simulink model "Scenario_1"  (R2020b)
settings: Solver=ode1  StartTime=0.0  StopTime=10  FixedStep=Ts  RelTol=1e-3
InitFcn:
  | Scenario_1_parameters;
values from neighbouring files (symbols this model uses):
  c0 = c0_zeb    (= 6.57988e-09)    [Scenario_17_parameters.m]    (also in Scenario_1_parameters.m = 6.37282e-09; Scenario_2_parameters.m = 6.37282e-09; Scenario_3_parameters.m)
  c1 = c1_zeb    (= 9.15905e-09)    [Scenario_17_parameters.m]    (also in Scenario_1_parameters.m = 8.76156e-09; Scenario_2_parameters.m = 8.76156e-09; Scenario_3_parameters.m)
  fg = 50    [Scenario_17_parameters.m]    (also in Scenario_1_parameters.m; Scenario_2_parameters.m; Scenario_3_parameters.m)
  G1gen = 0.50    (= 0.5)    [Scenario_17_parameters.m]    (also in Scenario_1_parameters.m = 0.2; Scenario_2_parameters.m = 0.1245; Scenario_3_parameters.m = 0.45)
  G2gen = 0.30    (= 0.3)    [Scenario_1_parameters.m]    (also in Scenario_2_parameters.m; Scenario_3_parameters.m = 0.4)
  G3gen = 0.25    [Scenario_1_parameters.m]    (also in Scenario_2_parameters.m = 0.2; Scenario_3_parameters.m = 0.6)
  G5gen = 0.75    [Scenario_17_parameters.m]    (also in Scenario_1_parameters.m = 0.22; Scenario_2_parameters.m = 0.2; Scenario_3_parameters.m = 0.7)
  G6gen = 0.90    (= 0.9)    [Scenario_17_parameters.m]    (also in Scenario_1_parameters.m = 0.41; Scenario_2_parameters.m = 0.2078; Scenario_3_parameters.m = 0.95)
  G7gen = 0.60    (= 0.6)    [Scenario_17_parameters.m]    (also in Scenario_1_parameters.m = 0.52; Scenario_2_parameters.m = 0.518; Scenario_3_parameters.m = 0.5)
  Ihvpk = Ihv*sqrt(2)    [Scenario_17_parameters.m]    (also in Scenario_1_parameters.m; Scenario_2_parameters.m; Scenario_3_parameters.m)
  l0 = l0_zeb    (= 0.00368)    [Scenario_17_parameters.m]    (also in Scenario_1_parameters.m = 0.00373; Scenario_2_parameters.m = 0.00373; Scenario_3_parameters.m)
  l1 = l1_zeb    (= 0.00128)    [Scenario_17_parameters.m]    (also in Scenario_1_parameters.m = 0.00133; Scenario_2_parameters.m = 0.00133; Scenario_3_parameters.m)
  L3dem = 0.30    (= 0.3)    [Scenario_17_parameters.m]    (also in Scenario_1_parameters.m = 0.1; Scenario_2_parameters.m = 0.1; Scenario_3_parameters.m = 0.2)
  L4dem = 0.30    (= 0.3)    [Scenario_1_parameters.m]    (also in Scenario_2_parameters.m)
  L5dem = 0.25    [Scenario_17_parameters.m]    (also in Scenario_1_parameters.m = 0.35; Scenario_2_parameters.m = 0.35)
  L6dem = 0.15    [Scenario_1_parameters.m]    (also in Scenario_2_parameters.m; Scenario_3_parameters.m = 0.1)
  L7dem = 0.10    (= 0.1)    [Scenario_1_parameters.m]    (also in Scenario_2_parameters.m; Scenario_3_parameters.m = 0.15)
  Pr = Sr*PF    (= 1900000000)    [Scenario_17_parameters.m]    (also in Scenario_1_parameters.m = 550050000; Scenario_2_parameters.m = 550050000; Scenario_3_parameters.m = 11640000000)
  Qr = sqrt(Sr^2 - Pr^2)    [Scenario_17_parameters.m]    (also in Scenario_1_parameters.m; Scenario_2_parameters.m; Scenario_3_parameters.m)
  r0 = r0_zeb    (= 0.39362)    [Scenario_17_parameters.m]    (also in Scenario_1_parameters.m = 0.44587; Scenario_2_parameters.m = 0.44587; Scenario_3_parameters.m)
  r1 = r1_zeb    (= 0.06862)    [Scenario_17_parameters.m]    (also in Scenario_1_parameters.m = 0.12087; Scenario_2_parameters.m = 0.12087; Scenario_3_parameters.m)
  Rtpu = Xtpu/40    (= 0.0025)    [Scenario_17_parameters.m]    (also in Scenario_1_parameters.m = 0.00375; Scenario_2_parameters.m = 0.00375; Scenario_3_parameters.m = 0.00375)
  S1non = 700e6    (= 700000000)    [Scenario_17_parameters.m]    (also in Scenario_1_parameters.m = 400000000; Scenario_2_parameters.m = 400000000; Scenario_3_parameters.m = 1000000000)
  S2non = 300e6    (= 300000000)    [Scenario_1_parameters.m]    (also in Scenario_2_parameters.m; Scenario_3_parameters.m = 3000000000)
  S3non = 200e6    (= 200000000)    [Scenario_1_parameters.m]    (also in Scenario_2_parameters.m; Scenario_3_parameters.m = 1000000000)
  S5non = 400e6    (= 400000000)    [Scenario_17_parameters.m]    (also in Scenario_1_parameters.m = 500000000; Scenario_2_parameters.m = 500000000; Scenario_3_parameters.m = 2000000000)
  S6non = 150e6    (= 150000000)    [Scenario_17_parameters.m]    (also in Scenario_1_parameters.m = 400000000; Scenario_2_parameters.m = 400000000; Scenario_3_parameters.m = 3000000000)
  S7non = 1000e6    (= 1000000000)    [Scenario_17_parameters.m]    (also in Scenario_1_parameters.m = 200000000; Scenario_2_parameters.m = 200000000; Scenario_3_parameters.m = 4000000000)
  tonvsc = 0.01    [Scenario_17_parameters.m]    (also in Scenario_1_parameters.m = 0.02; Scenario_2_parameters.m; Scenario_3_parameters.m = 0.05)
  Ts = 100e-6    (= 0.0001)    [Scenario_17_parameters.m]    (also in Scenario_1_parameters.m; Scenario_2_parameters.m; Scenario_3_parameters.m = 5e-05)
  Vhv = 220e3    (= 220000)    [Scenario_17_parameters.m]    (also in Scenario_1_parameters.m; Scenario_2_parameters.m; Scenario_3_parameters.m)
  Vmv = 22e3    (= 22000)    [Scenario_17_parameters.m]    (also in Scenario_1_parameters.m; Scenario_2_parameters.m; Scenario_3_parameters.m)
  wc1 = wsw1/10    (= 848.230016469)    [Scenario_17_parameters.m]    (also in Scenario_1_parameters.m; Scenario_2_parameters.m; Scenario_3_parameters.m)
  wdc1 = wc1/10    (= 84.8230016469)    [Scenario_17_parameters.m]    (also in Scenario_1_parameters.m; Scenario_2_parameters.m; Scenario_3_parameters.m)
  wpq1 = wc1/10    (= 84.8230016469)    [Scenario_17_parameters.m]    (also in Scenario_1_parameters.m; Scenario_2_parameters.m; Scenario_3_parameters.m)
  wsw1 = ksw1*2*pi*fg    (= 8482.30016469)    [Scenario_17_parameters.m]    (also in Scenario_1_parameters.m; Scenario_2_parameters.m; Scenario_3_parameters.m)
  Xtpu = 0.10    (= 0.1)    [Scenario_17_parameters.m]    (also in Scenario_1_parameters.m = 0.15; Scenario_2_parameters.m = 0.15; Scenario_3_parameters.m = 0.15)
undefined symbols (not defined in the file or in its folder): D11, Delta, Kf, r, theta0
libraries: powerlib x206, simulink_extras x140, powerlib_meascontrol x82, pid_lib x48, eeGeneralControl x32, simulink x28, eeTransforms x24, spsFirstOrderFilterLib x16, eePwmGeneratorTwoLevel x4
(part 3 of 16)

== system Scenario_1/G6 ==
  Bus Selector : BusSelector  OutputSignals=Pabc,Qabc,vqp,vdp,vqn,vdn,iqp,idp,iqn,idn,f
  Goto1 : Goto  Commented=on  GotoTag=Pg6  TagVisibility=global
  Goto5 : Goto  Commented=on  GotoTag=Qg6  TagVisibility=global
  Mux2 : Mux
  Mux3 : Mux
  VSC : Subsystem  mask{vscmod=Phasor I-ref, fg=fg, Vhv=Vhv, Vmv=Vmv, Pconv=100e6, Rtpu=Rtpu, Xtpu=Xtpu, Hvsc=30e-3, qmode=Active power, dmode=Reactive power, wsw=wsw1, wn_pll=2*pi*80, wc=wc1, wpq=wpq1, wdc=wdc1, koc=1.2, tfilt=1*(1/wsw1), negseq_en=off, fdroop_en=on, Vacdroop_en=on, LVRT_en=on, Kfdroop=0.05, Kvdroop=0.1, Vlvrt0=0.9, Vlvrt_min=0.5, Qmax_lvrt=0.9}
      mask prompts: vscmod "VSC Model"; fg "AC grid frequency (Hz)"; Vhv "Grid-side voltage (V)(LL-rms)"; Vmv "Converter-side voltage (V)(LL-rms)"; Pconv "Converter nominal power (VA)"; Rtpu "Resistance seen by the converter (p.u)"; Xtpu "Reactance seen by the converter (p.u)"; Hvsc "VSC equivalent inertia (s)"; qmode "q-axis control mode"; dmode "d-axis control mode"; wsw "Switching frequency (rad/s)"; wn_pll "PLL filter natural frequency"; wc "Current-control bandwidth (rad/s)"; wpq "PQ control bandwidth (rad/s)"; wdc "DC Voltage control bandwidth(rad/s)"; koc "Overcurrent factor (p.u)"; tfilt "Vabc filter time constant (s)"; negseq_en "Enable negative sequence control"; fdroop_en "Enable frequency droop"; Vacdroop_en "Enable AC voltage droop"; LVRT_en "Enable LVRT"; Kfdroop "Frequency droop (p.u)"; Kvdroop "Voltage droop (p.u)"; Vlvrt0 "initial voltage (p.u)"; Vlvrt_min "minimum voltage (p.u)"; Qmax_lvrt "max power injected at min voltage (p.u)"
      mask init: same as Scenario_1/G2/VSC
      mask TypeOptions vscmod: EMT Switching | EMT Average | Phasor Quasi-EMT | Phasor I-1st | Phasor I-ref | Phasor PQ-1st
      mask Callback vscmod:
      | % Control parameter visiblity
      | 
      | % Get the value of the Enable Bias checkbox
      | % unchecked = 'off'
      | % checked = 'on'
      | 
      | maskObj = Simulink.Mask.get(gcb);
      | 
      | wn_pll = 'on';
      | wsw = 'on';
      | vscmod = get_param(gcb,'vscmod');
      |     if strcmp(vscmod,'EMT Switching')
      |       wn_pll = 'on';
      |       wsw = 'on';
      |       tfilt = 'on';
      |     elseif strcmp(vscmod,'EMT Average')
      |         wn_pll = 'on';
      |         wsw = 'off';
      |         tfilt = 'off';
      |     elseif strcmp(vscmod,'Phasor Quasi-EMT')
      |         wn_pll = 'off';
      |         wsw = 'off';
      |         tfilt = 'off';
      |     elseif strcmp(vscmod,'Phasor I-1st')
      |         wn_pll = 'off';
      |         wsw = 'off';
      |         tfilt = 'off';
      |     elseif strcmp(vscmod,'Phasor I-ref')
      |         wn_pll = 'off';
      |         wsw = 'off';
      |         tfilt = 'off';
      |     elseif strcmp(vscmod,'Phasor PQ-1st')
      |         wn_pll = 'off';
      |         wsw = 'off';
      |         tfilt = 'off';
      |     end
      | 
      | fdroop_en = get_param(gcb,'fdroop_en');
      | Vacdroop_en = get_param(gcb,'Vacdroop_en');
      | LVRT_en = get_param(gcb,'LVRT_en');
      | negseq_en = get_param(gcb,'negseq_en');
      | 
      | % Set the 'MaskVisibilities' property for each parameters
      |     set_param(gcb,'MaskVisibilities',{'on','on','on','on','on','on','on','on','on','on',wsw,wn_pll,'on','on','on','on',tfilt,'on','on','on','on',fdroop_en,Vacdroop_en,'on','on','on'});
      | 
      | % Make LVRT area visible when it is enabled
      | if strcmp(LVRT_en,'on')
      |   maskObj.getDialogControl('Container_LVRT').Visible = 'on';
      | else
      |     maskObj.getDialogControl('Container_LVRT').Visible = 'off';
      | end
      | 
      | % Note that the value of the bias is not handled here.
      | % See the Initialization tab
      mask TypeOptions qmode: Active power | DC voltage
      mask Callback qmode:
      | %if strcmp(qmode,'Active Power')
      | %    disp(qmode)
      | %elseif strcmp(qmode,'DC Voltage')
      | %    disp(qmode)
      | %end
      mask TypeOptions dmode: Reactive power | AC voltage
      mask Callback fdroop_en:
      | % Control parameter visiblity
      | 
      | % Get the value of the Enable Bias checkbox
      | % unchecked = 'off'
      | % checked = 'on'
      | 
      | maskObj = Simulink.Mask.get(gcb);
      | 
      | wn_pll = 'on';
      | wsw = 'on';
      | vscmod = get_param(gcb,'vscmod');
      |     if strcmp(vscmod,'EMT Switching')
      |       wn_pll = 'on';
      |       wsw = 'on';
      |       tfilt = 'on';
      |     elseif strcmp(vscmod,'EMT Average')
      |         wn_pll = 'on';
      |         wsw = 'off';
      |         tfilt = 'off';
      |     elseif strcmp(vscmod,'Phasor Quasi-EMT')
      |         wn_pll = 'off';
      |         wsw = 'off';
      |         tfilt = 'off';
      |     elseif strcmp(vscmod,'Phasor I-1st')
      |         wn_pll = 'off';
      |         wsw = 'off';
      |         tfilt = 'off';
      |     elseif strcmp(vscmod,'Phasor I-ref')
      |         wn_pll = 'off';
      |         wsw = 'off';
      |         tfilt = 'off';
      |     elseif strcmp(vscmod,'Phasor PQ-1st')
      |         wn_pll = 'off';
      |         wsw = 'off';
      |         tfilt = 'off';
      |     end
      | 
      | fdroop_en = get_param(gcb,'fdroop_en');
      | Vacdroop_en = get_param(gcb,'Vacdroop_en');
      | LVRT_en = get_param(gcb,'LVRT_en');
      | negseq_en = get_param(gcb,'negseq_en');
      | 
      | % Set the 'MaskVisibilities' property for each parameters
      |     set_param(gcb,'MaskVisibilities',{'on','on','on','on','on','on','on','on','on','on',wsw,wn_pll,'on','on','on','on',tfilt,'on','on','on','on',fdroop_en,Vacdroop_en,'on','on','on'});
      | 
      | % Make LVRT area visible when it is enabled
      | if strcmp(LVRT_en,'on')
      |   maskObj.getDialogControl('Container_LVRT').Visible = 'on';
      | else
      |     maskObj.getDialogControl('Container_LVRT').Visible = 'off';
      | end
      | 
      | % Note that the value of the bias is not handled here.
      | % See the Initialization tab
      mask Callback Vacdroop_en:
      | % Control parameter visiblity
      | 
      | % Get the value of the Enable Bias checkbox
      | % unchecked = 'off'
      | % checked = 'on'
      | 
      | maskObj = Simulink.Mask.get(gcb);
      | 
      | wn_pll = 'on';
      | wsw = 'on';
      | vscmod = get_param(gcb,'vscmod');
      |     if strcmp(vscmod,'EMT Switching')
      |       wn_pll = 'on';
      |       wsw = 'on';
      |       tfilt = 'on';
      |     elseif strcmp(vscmod,'EMT Average')
      |         wn_pll = 'on';
      |         wsw = 'off';
      |         tfilt = 'off';
      |     elseif strcmp(vscmod,'Phasor Quasi-EMT')
      |         wn_pll = 'off';
      |         wsw = 'off';
      |         tfilt = 'off';
      |     elseif strcmp(vscmod,'Phasor I-1st')
      |         wn_pll = 'off';
      |         wsw = 'off';
      |         tfilt = 'off';
      |     elseif strcmp(vscmod,'Phasor I-ref')
      |         wn_pll = 'off';
      |         wsw = 'off';
      |         tfilt = 'off';
      |     elseif strcmp(vscmod,'Phasor PQ-1st')
      |         wn_pll = 'off';
      |         wsw = 'off';
      |         tfilt = 'off';
      |     end
      | 
      | fdroop_en = get_param(gcb,'fdroop_en');
      | Vacdroop_en = get_param(gcb,'Vacdroop_en');
      | LVRT_en = get_param(gcb,'LVRT_en');
      | negseq_en = get_param(gcb,'negseq_en');
      | 
      | % Set the 'MaskVisibilities' property for each parameters
      |     set_param(gcb,'MaskVisibilities',{'on','on','on','on','on','on','on','on','on','on',wsw,wn_pll,'on','on','on','on',tfilt,'on','on','on','on',fdroop_en,Vacdroop_en,'on','on','on'});
      | 
      | % Make LVRT area visible when it is enabled
      | if strcmp(LVRT_en,'on')
      |   maskObj.getDialogControl('Container_LVRT').Visible = 'on';
      | else
      |     maskObj.getDialogControl('Container_LVRT').Visible = 'off';
      | end
      | 
      | % Note that the value of the bias is not handled here.
      | % See the Initialization tab
      mask Callback LVRT_en:
      | % Control parameter visiblity
      | 
      | % Get the value of the Enable Bias checkbox
      | % unchecked = 'off'
      | % checked = 'on'
      | 
      | maskObj = Simulink.Mask.get(gcb);
      | 
      | wn_pll = 'on';
      | wsw = 'on';
      | vscmod = get_param(gcb,'vscmod');
      |     if strcmp(vscmod,'EMT Switching')
      |       wn_pll = 'on';
      |       wsw = 'on';
      |       tfilt = 'on';
      |     elseif strcmp(vscmod,'EMT Average')
      |         wn_pll = 'on';
      |         wsw = 'off';
      |         tfilt = 'off';
      |     elseif strcmp(vscmod,'Phasor Quasi-EMT')
      |         wn_pll = 'off';
      |         wsw = 'off';
      |         tfilt = 'off';
      |     elseif strcmp(vscmod,'Phasor I-1st')
      |         wn_pll = 'off';
      |         wsw = 'off';
      |         tfilt = 'off';
      |     elseif strcmp(vscmod,'Phasor I-ref')
      |         wn_pll = 'off';
      |         wsw = 'off';
      |         tfilt = 'off';
      |     elseif strcmp(vscmod,'Phasor PQ-1st')
      |         wn_pll = 'off';
      |         wsw = 'off';
      |         tfilt = 'off';
      |     end
      | 
      | fdroop_en = get_param(gcb,'fdroop_en');
      | Vacdroop_en = get_param(gcb,'Vacdroop_en');
      | LVRT_en = get_param(gcb,'LVRT_en');
      | negseq_en = get_param(gcb,'negseq_en');
      | 
      | % Set the 'MaskVisibilities' property for each parameters
      |     set_param(gcb,'MaskVisibilities',{'on','on','on','on','on','on','on','on','on','on',wsw,wn_pll,'on','on','on','on',tfilt,'on','on','on','on',fdroop_en,Vacdroop_en,'on','on','on'});
      | 
      | % Make LVRT area visible when it is enabled
      | if strcmp(LVRT_en,'on')
      |   maskObj.getDialogControl('Container_LVRT').Visible = 'on';
      | else
      |     maskObj.getDialogControl('Container_LVRT').Visible = 'off';
      | end
      | 
      | % Note that the value of the bias is not handled here.
      | % See the Initialization tab
      mask DialogControl DescTextVar Prompt: Three-phase VSC model
      mask DialogControl Tab1 Prompt: Electrical parameters
      mask DialogControl Tab2 Prompt: Control parameters
      mask DialogControl Tab3 Prompt: Other parameters
      mask DialogControl Container_LVRT Prompt: LVRT
      mask Display:
      | choice = get_param(gcb,'vscmod');
      | if strcmp(choice,'Phasor Quasi-EMT')
      |     disp('VSC\n\n')
      |     disp('\n\nPhasor\n\n')
      |     disp('\n\nQuasi-EMT')
      | elseif strcmp(choice,'EMT Average')
      |     disp('VSC\n')
      |     disp('\nEMT AVG')
      | elseif strcmp(choice,'EMT Switching')
      |     disp('VSC\n')
      |     disp('\nEMT SW')
      | elseif strcmp(choice,'Phasor I-1st')
      |     disp('VSC\n\n')
      |     disp('\n\nPhasor\n\n')
      |     disp('\n\nI 1st')
      | elseif strcmp(choice,'Phasor I-ref')
      |     disp('VSC\n\n')
      |     disp('\n\nPhasor\n\n')
      |     disp('\n\nI ref')
      | elseif strcmp(choice,'Phasor PQ-1st')
      |     disp('VSC\n\n')
      |     disp('\n\nPhasor\n\n')
      |     disp('\n\nPQ 1st')
      | end
  A : PMIOPort  Side=Right
  B : PMIOPort  Port=2  Side=Right
  C : PMIOPort  Port=3  Side=Right
  tag scope: fg6=global, idqpng6=global, vdqpng6=global
  wires:
  Bus Selector/9 -> Mux3/3  "<iqn>"
  Bus Selector/3 -> Mux2/1  "<vqp>"
  Bus Selector/4 -> Mux2/2  "<vdp>"
  Bus Selector/1 -> Goto1/1  "<Pabc>"
  Bus Selector/8 -> Mux3/2  "<idp>"
  Mux3/1 -> [idqpng6]
  Bus Selector/10 -> Mux3/4  "<idn>"
  Mux2/1 -> [vdqpng6]
  Bus Selector/6 -> Mux2/4  "<vdn>"
  Bus Selector/7 -> Mux3/1  "<iqp>"
  VSC/1(m) -> Bus Selector/1
  Bus Selector/5 -> Mux2/3  "<vqn>"
  Bus Selector/11 -> [fg6]  "<f>"
  Bus Selector/2 -> Goto5/1  "<Qabc>"
  connections:
  VSC/LConn2 -- B/RConn1
  VSC/LConn1 -- A/RConn1
  VSC/LConn3 -- C/RConn1

== system Scenario_1/G7 ==
  note: Synchronous Machine Model according to ENTSO-E
  note: Nomenclature (according to IEEE Std 421.1-2007):
      | Efd = Exciter output voltage (generator field voltage)
      | Ifd = Exciter output current (generator field current)
      | Vf = Excitation system stabilizer signal
      | Vfe = Signal proportional to exciter field current
      | Vl = Limiters and protective elements feedback
      | Vr = Regulator output
      | Vs = Power System Stabilizer (PSS) output
      | Vsi = Power System Stabilizer (PSS) inputs (shaft speed, frequency, generator electric power, and others
      | Vt = Generator terminal voltage
      | It = Generator terminal current
      | Vref = Voltage regulator reference signal
      | Vc = terminal voltage transducer output
  Bus Selector : BusSelector  OutputSignals=dw,w,vq,vd,iq,id,Peo,Te
  Constant : Constant  Value=G7gen
  Exciter System : Subsystem
  Real-Imag to Complex : RealImagToComplex
  Real-Imag to Complex1 : RealImagToComplex
  Ref voltage (p.u) : Constant  Value=1.0 + 5e-3
  Snubber : powerlib/Elements/Three-Phase Parallel RLC Load  LConnTagsString=A|B|C  Configuration=Y (grounded)  NominalVoltage=Vmv  Vabc=[1e3 1e3 1e3]  Vabcp=[1e3 1e3 1e3]  NominalFrequency=fg  UnbalancedPower=off  ActivePower=S7non*0.01  InductivePower=0  CapacitivePower=0  Pabc=[10e3 9e3 11e3]  QLabc=[100 90 110]  QCabc=[100 90 110]  Pabcp=[10e3 9e3 11e3]  QLabcp=[100 90 110]  QCabcp=[100 90 110]  Measurements=None  LoadType=constant Z
  Speed Governor : Subsystem  mask{R=0.05, T1=0.5, T2=3, T3=10, Dt=0, Vmin=0, Vmax=10, P0=G7gen}
      mask prompts: R "Controller droop (R)"; T1 "Governor time constant (T1)(sec)"; T2 "Turbine derivative time constant (T2)(sec)"; T3 "Turbine delay time constant (T3)(sec)"; Dt "Frictional losses factor (Dt)"; Vmin "Minimum gate limit (Vmin)(p.u)"; Vmax "Maximum gate limit (Vmax)(p.u)"; P0 "Initial power (p.u)"
      mask Display:
      | disp('TGOV')
      | 
      | port_label('input',1,'Pref')
      | port_label('input',2,'dw')
      | 
      | port_label('output',1,'Pm')
  Synchronous Machine pu Standard : powerlib/Machines/Synchronous Machine pu Standard  PresetModel=No  MechanicalLoad=Mechanical power Pm  ShowDetailedParameters=on  RotorType=Salient-pole  Units=per unit standard parameters  MeasurementBus=on  NominalParameters=[S7non Vmv fg]  Reactances1=[ 1.81, 0.3, 0.23, 1.76, 0.65, 0.25, 0.15 ]  Reactances2=[1.667 0.25 0.2333 1.125 0.225 0.15]  dAxisTimeConstants=Open-circuit  qAxisTimeConstants=Open-circuit  TimeConstants1="[6  0.002  0.002]"  TimeConstants2=[ 8.0, 0.03, 1.0, 0.07 ]  TimeConstants3="[  4.49  0.0681  0.0513  ]"  TimeConstants4=[ 8.0, 0.03, 0.3371, 0.0295 ]  TimeConstants5=[ 1.01, 0.053, 0.1 ]  TimeConstants6=[ 1.3201, 0.023, 1.0, 0.07 ]  TimeConstants7=[0.012 0.003 0.003]  TimeConstants8=[ 1.3201, 0.0231, 0.3371, 0.0295 ]  StatorResistance=0.01  Mechanical=[3 0 2]  PolePairs=20  InitialConditions=[0 -74.7064 0.607738 0.607738 0.607738 -41.2057 -161.206 78.7943 1.5]  SetSaturation=off  Saturation=[0.6404,0.7127,0.8441,0.9214,0.9956,1.082,1.19,1.316,1.457;0.7,0.7698,0.8872,0.9466,0.9969,1.046,1.1,1.151,1.201]  LoadFlowParameters=[1 100000000 0 0 0]  TsPowergui=0  TsBlock=-1  IterativeModel=Trapezoidal non iterative  IterativeDiscreteModel=Trapezoidal non iterative  BusType=PV  Pref=S7non*G7gen  Qref=0  Qmin=-inf  Qmax=inf  PLF=0  QLF=0
  Three-Phase Transformer (Two Windings) : powerlib/Elements/Three-Phase Transformer (Two Windings)  Winding1Connection=Delta (D11)  Winding2Connection=Yg  CoreType=Three single-phase transformers  SetSaturation=off  Hysteresis=off  DataFile='hysteresis'  SetInitialFlux=off  Measurements=None  UNITS=pu  NominalPower=[S7non , fg ]  Winding1=[Vmv 0.00125 0.05]  Winding2=[Vhv 0.00125 0.05]  Rm=5000  Lm=5000  L0=0.5  Saturation=[ 0,0 ; 0.0024,1.2 ; 1.0,1.52 ]  InitialFluxes=[ 0.8 , -0.8 , 0.7 ]  BreakLoop=off  DiscreteSolver=Trapezoidal iterative  DataType=off  TransfoNumber=1
  Transfer Fcn (with initial outputs) : simulink_extras/Additional Linear/Transfer Fcn (with initial outputs)  Commented=on  N=[-1.8]  D="[1  0]"  Y0=0.0705  U0=0
  A : PMIOPort  Side=Right
  B : PMIOPort  Port=2  Side=Right
  C : PMIOPort  Port=3  Side=Right
  tag scope: Pe7=global, Te7=global, wm7=global
  wires:
  Ref voltage (p.u)/1 -> Exciter System/2(Vref)
  Bus Selector/1 -> Speed Governor/2(dw), Exciter System/1(<dw>)  "<dw>"
  Bus Selector/4 -> Real-Imag to Complex/2  "<vd>"
  Bus Selector/3 -> Real-Imag to Complex/1  "<vq>"
  Bus Selector/5 -> Real-Imag to Complex1/1  "<iq>"
  Bus Selector/6 -> Real-Imag to Complex1/2  "<id>"
  Real-Imag to Complex/1 -> Exciter System/3(Vt)
  Real-Imag to Complex1/1 -> Exciter System/4(It)
  Bus Selector/7 -> [Pe7], Exciter System/5(<Peo>)  "<Peo>"
  Bus Selector/8 -> [Te7]  "<Te>"
  Speed Governor/1(Pm) -> Synchronous Machine pu Standard/1
  Exciter System/1(Efd) -> Synchronous Machine pu Standard/2
  Synchronous Machine pu Standard/1 -> Bus Selector/1
  Constant/1 -> Speed Governor/1(RefL)
  Bus Selector/2 -> [wm7]  "<w>"
  connections:
  Snubber/LConn1 -- Synchronous Machine pu Standard/RConn1 -- Three-Phase Transformer (Two Windings)/LConn1
  Snubber/LConn3 -- Synchronous Machine pu Standard/RConn3 -- Three-Phase Transformer (Two Windings)/LConn3
  Snubber/LConn2 -- Synchronous Machine pu Standard/RConn2 -- Three-Phase Transformer (Two Windings)/LConn2
  Three-Phase Transformer (Two Windings)/RConn1 -- A/RConn1
  Three-Phase Transformer (Two Windings)/RConn2 -- B/RConn1
  Three-Phase Transformer (Two Windings)/RConn3 -- C/RConn1

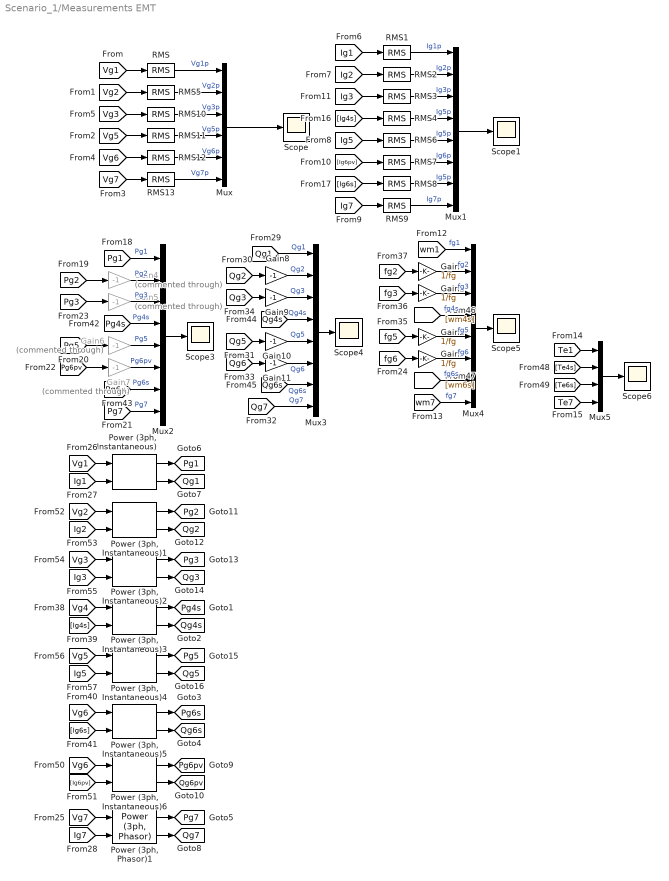
== system Scenario_1/Measurements EMT ==
  Gain{,1..3} (4 alike) : Gain  Gain=1/fg
  Gain{8..11} (4 alike) : Gain  Gain=-1
  Gain{4..7} (4 alike) : Gain  Commented=through  Gain=-1
  Mux : Mux  Inputs=6
  Mux{1..4} (4 alike) : Mux  Inputs=8
  Mux5 : Mux
  Power (3ph, Instantaneous){,1..6} (7 alike) : powerlib_meascontrol/Measurements/Power (3ph, Instantaneous)
  "Power (3ph, Phasor)1" : powerlib_meascontrol/Measurements/Power (3ph, Phasor)
      settings: SourceProductBaseCode=PS
  RMS{,1..13} (14 alike) : powerlib_meascontrol/Measurements/RMS  TrueRMS=on  Freq=fg  RMSInit=0  Ts=0
  Scope{,1,3..6} (6 alike) : Scope
  tag scope: Pg1=global, Pg2=global, Pg3=global, Pg4s=global, Pg5=global, Pg6pv=global, Pg6s=global, Pg7=global, Qg1=global, Qg2=global, Qg3=global, Qg4s=global, Qg5=global, Qg6pv=global, Qg6s=global, Qg7=global
  wires:
  "Power (3ph, Instantaneous)4"/1 -> [Pg5]
  [Ig5] -> "Power (3ph, Instantaneous)4"/2
  "Power (3ph, Instantaneous)4"/2 -> [Qg5]
  [Vg5] -> "Power (3ph, Instantaneous)4"/1
  [Ig3] -> "Power (3ph, Instantaneous)2"/2
  [Vg3] -> "Power (3ph, Instantaneous)2"/1
  "Power (3ph, Instantaneous)2"/1 -> [Pg3]
  "Power (3ph, Instantaneous)2"/2 -> [Qg3]
  [Vg2] -> "Power (3ph, Instantaneous)1"/1
  "Power (3ph, Instantaneous)1"/2 -> [Qg2]
  "Power (3ph, Instantaneous)1"/1 -> [Pg2]
  [Ig2] -> "Power (3ph, Instantaneous)1"/2
  "Power (3ph, Instantaneous)6"/1 -> [Pg6pv]
  [Ig6pv] -> "Power (3ph, Instantaneous)6"/2
  "Power (3ph, Instantaneous)6"/2 -> [Qg6pv]
  [Vg6] -> "Power (3ph, Instantaneous)6"/1
  [Te6s] -> Mux5/3
  [Te4s] -> Mux5/2
  [Te7] -> Mux5/4
  [wm6s] -> Mux4/7  "fg6s"
  [wm4s] -> Mux4/4  "fg4s"
  Gain2/1 -> Mux4/5  "fg5"
  Gain3/1 -> Mux4/6  "fg6"
  [wm7] -> Mux4/8  "fg7"
  [Qg6s] -> Mux3/7  "Qg6s"
  [Qg4s] -> Mux3/4  "Qg4s"
  Gain10/1 -> Mux3/5  "Qg5"
  Gain11/1 -> Mux3/6  "Qg6"
  [Qg7] -> Mux3/8  "Qg7"
  [Pg6s] -> Mux2/7  "Pg6s"
  [Pg4s] -> Mux2/4  "Pg4s"
  Gain6/1 -> Mux2/5  "Pg5"
  Gain7/1 -> Mux2/6  "Pg6pv"
  [Pg7] -> Mux2/8  "Pg7"
  "Power (3ph, Instantaneous)5"/2 -> [Qg6s]
  "Power (3ph, Instantaneous)5"/1 -> [Pg6s]
  [Ig6s] -> "Power (3ph, Instantaneous)5"/2
  [Vg6] -> "Power (3ph, Instantaneous)5"/1
  [Vg4] -> "Power (3ph, Instantaneous)3"/1
  [Ig4s] -> "Power (3ph, Instantaneous)3"/2
  "Power (3ph, Instantaneous)3"/1 -> [Pg4s]
  "Power (3ph, Instantaneous)3"/2 -> [Qg4s]
  RMS8/1 -> Mux1/7  "Ig5p"
  [Ig6s] -> RMS8/1
  RMS4/1 -> Mux1/4  "Ig5p"
  [Ig4s] -> RMS4/1
  RMS9/1 -> Mux1/8  "Ig7p"
  RMS7/1 -> Mux1/6  "Ig6p"
  RMS6/1 -> Mux1/5  "Ig5p"
  Gain9/1 -> Mux3/3  "Qg3"
  [Qg6] -> Gain11/1
  [Qg5] -> Gain10/1
  [Qg3] -> Gain9/1
  Gain8/1 -> Mux3/2  "Qg2"
  [Qg2] -> Gain8/1
  Gain5/1 -> Mux2/3  "Pg3"
  Gain4/1 -> Mux2/2  "Pg2"
  Mux5/1 -> Scope6/1
  [Te1] -> Mux5/1
  [fg6] -> Gain3/1
  [fg5] -> Gain2/1
  Gain1/1 -> Mux4/3  "fg3"
  [fg3] -> Gain1/1
  Gain/1 -> Mux4/2  "fg2"
  [fg2] -> Gain/1
  [wm1] -> Mux4/1  "fg1"
  Mux4/1 -> Scope5/1
  [Qg1] -> Mux3/1  "Qg1"
  Mux3/1 -> Scope4/1
  [Pg6pv] -> Gain7/1
  [Pg5] -> Gain6/1
  [Pg3] -> Gain5/1
  [Pg2] -> Gain4/1
  "Power (3ph, Phasor)1"/2 -> [Qg7]
  "Power (3ph, Instantaneous)"/2 -> [Qg1]
  "Power (3ph, Phasor)1"/1 -> [Pg7]
  "Power (3ph, Instantaneous)"/1 -> [Pg1]
  [Ig7] -> "Power (3ph, Phasor)1"/2
  [Vg7] -> "Power (3ph, Phasor)1"/1
  [Ig1] -> "Power (3ph, Instantaneous)"/2
  [Vg1] -> "Power (3ph, Instantaneous)"/1
  Mux1/1 -> Scope1/1
  [Ig7] -> RMS9/1
  [Ig6pv] -> RMS7/1
  [Ig5] -> RMS6/1
  RMS3/1 -> Mux1/3  "Ig3p"
  [Ig3] -> RMS3/1
  RMS2/1 -> Mux1/2  "Ig2p"
  [Ig2] -> RMS2/1
  RMS1/1 -> Mux1/1  "Ig1p"
  [Ig1] -> RMS1/1
  Mux/1 -> Scope/1
  RMS13/1 -> Mux/6  "Vg7p"
  [Vg7] -> RMS13/1
  RMS12/1 -> Mux/5  "Vg6p"
  [Vg6] -> RMS12/1
  RMS11/1 -> Mux/4  "Vg5p"
  [Vg5] -> RMS11/1
  RMS10/1 -> Mux/3  "Vg3p"
  [Vg3] -> RMS10/1
  RMS5/1 -> Mux/2  "Vg2p"
  [Vg2] -> RMS5/1
  RMS/1 -> Mux/1  "Vg1p"
  [Vg1] -> RMS/1
  [Pg1] -> Mux2/1  "Pg1"
  Mux2/1 -> Scope3/1

== system Scenario_1/Measurements Phasor ==
  Abs : Abs
  Gain{,1..3} (4 alike) : Gain  Gain=1/fg
  Gain{8..11} (4 alike) : Gain  Gain=-1
  Mux{,2..4} (4 alike) : Mux  Inputs=6
  Power (3ph, Phasor){,1,4..7} (6 alike) : powerlib_meascontrol/Measurements/Power (3ph, Phasor)
      settings: SourceProductBaseCode=PS
  Scope{,3..5} (4 alike) : Scope
  Subsystem1 : Subsystem
      mask init:
      | a = exp(1i*2*pi/3);
      | a2 = exp(1i*4*pi/3);
  Subsystem2 : Subsystem
      mask init:
      | a = exp(1i*2*pi/3);
      | a2 = exp(1i*4*pi/3);
  Subsystem3 : Subsystem
      mask init:
      | a = exp(1i*2*pi/3);
      | a2 = exp(1i*4*pi/3);
  Subsystem4 : Subsystem
      mask init:
      | a = exp(1i*2*pi/3);
      | a2 = exp(1i*4*pi/3);
  Subsystem5 : Subsystem
      mask init:
      | a = exp(1i*2*pi/3);
      | a2 = exp(1i*4*pi/3);
  Subsystem6 : Subsystem
      mask init:
      | a = exp(1i*2*pi/3);
      | a2 = exp(1i*4*pi/3);
  tag scope: Pg1=global, Pg2=global, Pg3=global, Pg5=global, Pg6=global, Pg7=global, Qg1=global, Qg2=global, Qg3=global, Qg5=global, Qg6=global, Qg7=global
  wires:
  Mux2/1 -> Scope3/1
  [Pg1] -> Mux2/1  "Pg1"
  [Vg1] -> Subsystem3/1(abc)
  Subsystem3/1(seq+) -> Mux/1  "Vg1p"
  [Vg2] -> Subsystem1/1(abc)
  Subsystem1/1(seq+) -> Mux/2  "Vg2p"
  [Vg3] -> Subsystem2/1(abc)
  Subsystem2/1(seq+) -> Mux/3  "Vg3p"
  [Vg5] -> Subsystem4/1(abc)
  Subsystem4/1(seq+) -> Mux/4  "Vg5p"
  [Vg6] -> Subsystem5/1(abc)
  Subsystem5/1(seq+) -> Mux/5  "Vg6p"
  [Vg7] -> Subsystem6/1(abc)
  Subsystem6/1(seq+) -> Mux/6  "Vg7p"
  [Vg1] -> "Power (3ph, Phasor)"/1
  [Ig1] -> "Power (3ph, Phasor)"/2
  [Vg7] -> "Power (3ph, Phasor)1"/1
  [Ig7] -> "Power (3ph, Phasor)1"/2
  "Power (3ph, Phasor)"/1 -> [Pg1]
  "Power (3ph, Phasor)1"/1 -> [Pg7]
  "Power (3ph, Phasor)"/2 -> [Qg1]
  "Power (3ph, Phasor)1"/2 -> [Qg7]
  Mux3/1 -> Scope4/1
  [Qg1] -> Mux3/1  "Qg1"
  Mux4/1 -> Scope5/1
  [wm1] -> Mux4/1  "fg1"
  [fg2] -> Gain/1
  Gain/1 -> Mux4/2  "fg2"
  [fg3] -> Gain1/1
  Gain1/1 -> Mux4/3  "fg3"
  [fg5] -> Gain2/1
  [fg6] -> Gain3/1
  [Pg2] -> Mux2/2  "Pg2"
  [Pg3] -> Mux2/3  "Pg3"
  [Qg2] -> Gain8/1
  Gain8/1 -> Mux3/2  "Qg2"
  [Qg3] -> Gain9/1
  [Qg5] -> Gain10/1
  [Qg6] -> Gain11/1
  Gain9/1 -> Mux3/3  "Qg3"
  [Vg6] -> "Power (3ph, Phasor)4"/1
  "Power (3ph, Phasor)4"/2 -> [Qg6]
  [Ig6] -> "Power (3ph, Phasor)4"/2
  "Power (3ph, Phasor)4"/1 -> [Pg6]
  [Ig2] -> "Power (3ph, Phasor)5"/2
  "Power (3ph, Phasor)5"/1 -> [Pg2]
  "Power (3ph, Phasor)5"/2 -> [Qg2]
  [Vg2] -> "Power (3ph, Phasor)5"/1
  "Power (3ph, Phasor)6"/2 -> [Qg3]
  "Power (3ph, Phasor)6"/1 -> [Pg3]
  [Vg3] -> "Power (3ph, Phasor)6"/1
  [Ig3] -> "Power (3ph, Phasor)6"/2
  [Vg5] -> "Power (3ph, Phasor)7"/1
  "Power (3ph, Phasor)7"/2 -> [Qg5]
  [Ig5] -> "Power (3ph, Phasor)7"/2
  "Power (3ph, Phasor)7"/1 -> [Pg5]
  [Pg5] -> Mux2/4  "Pg5"
  [Pg6] -> Mux2/5  "Pg6"
  [Pg7] -> Mux2/6  "Pg7"
  Gain10/1 -> Mux3/4  "Qg5"
  Gain11/1 -> Mux3/5  "Qg6"
  [Qg7] -> Mux3/6  "Qg7"
  Gain2/1 -> Mux4/4  "fg5"
  Gain3/1 -> Mux4/5  "fg6"
  [wm7] -> Mux4/6  "fg7"
  Mux/1 -> Abs/1
  Abs/1 -> Scope/1

== system Scenario_1/G1/Exciter System ==
  <dw> : Inport
  Vref : Inport  Port=2
  Vt : Inport  Port=3
  It : Inport  Port=4
  <Peo> : Inport  Port=5
  PSS1 : Subsystem  mask{Ks1=20, Ks2=0.1564, Ks3=1, Tw1=2, Tw2=2, Tw3=2, Tw4=0, T1=0.25, T2=0.2, T3=0.15, T4=0.1, T6=0, T7=2, T8=0.5, T9=0.1, Vstmin=-0.10, Vstmax=0.10, N=0, M=0, IC1=1, IC2=3}
      mask prompts: Ks1 "PSS gain (Ks1)"; Ks2 "2nd signal transducer factor(Ks2)"; Ks3 "washouts coupling factor (Ks3)"; Tw1 "1st washout 1th time constant (Tw1)(sec)"; Tw2 "1st washout 2nd time constant (Tw2)(sec)"; Tw3 "2nd washout 1st time constant (Tw3)(sec)"; Tw4 "2nd washout 2nd time constant (Tw4)(sec)"; T1 "1st lead-lag derivative time constant (T1)(sec)"; T2 "1st lead-lag delay time constant(T2)(sec)"; T3 "2nd lead-lag derivative time constant(T3)(sec)"; T4 "2nd lead-lag delay time constant(T4)(sec)"; T6 "1st signal transducer time constant(T6)(sec)"; T7 "2nd signal transducer time constant(T7)(sec)"; T8 "ramp tracking filter deriv. time constant(T8)(sec)"; T9 "ramp tracking filter delay time constant(T9)(sec)"; Vstmin "controller minimum output(Vstmin)"; Vstmax "controller maximum output(Vstmax)"; N "ramp tracking filter (N)"; M "ramp tracking filter (M)"; IC1 "1st input selector (IC1)"; IC2 "2nd input selector (IC2)"
      mask Display:
      | disp('PSS2A')
      | 
      | port_label('input',1,'dw')
      | port_label('input',2,'Pg')
      | %port_label('input',3,'Vs')
      | 
      | port_label('output',1,'Vs')
  SEXS : Subsystem  mask{K=200, Ta=3, Tb=10, Te=0.05, Emin=-4, Emax=4, Vf0=1.04}
      mask prompts: K "Controller gain (K)"; Ta "Filter derivative time constant (Ta)(sec)"; Tb "Filter delay time (Tb)(sec)"; Te "Exciter time constant (Te)(sec)"; Emin "Controller minimum output (Emin)"; Emax "Controller maximum output (Emax)"; Vf0 "Initial output (p.u)"
      mask Display:
      | disp('AVR')
      | 
      | port_label('input',1,'Vref')
      | port_label('input',2,'Vc')
      | port_label('input',3,'Vs')
      | 
      | port_label('output',1,'Efd')
  TR and LC_test : Subsystem  mask{Tr=1e-3, Rc=0, Xc=0}
      mask prompts: Tr "Transducter filter time constant (Tr)(sec)"; Rc "Resistance to compensate (p.u)"; Xc "Reactance to compensate (p.u)"
      mask Display:
      | %disp('Transducer \n \n')
      | %disp('and \n')
      | %disp('Load compensation')
      | text(15,35, 'Transducer')
      | text(30,24, 'and')
      | text(15,14, 'Load comp')
      | 
      | port_label('input',1,'Vt')
      | port_label('input',2,'It')
      | 
      | port_label('output',1,'Vc')
  Efd : Outport
  wires:
  TR and LC_test/1(Vc) -> SEXS/2(Vc)
  Vref/1 -> SEXS/1(Vref)
  Vt/1 -> TR and LC_test/1(Vt)
  <dw>/1 -> PSS1/1(dw)
  <Peo>/1 -> PSS1/2(Pgen)
  PSS1/1(Vothsg) -> SEXS/3(Vs)
  It/1 -> TR and LC_test/2(It)
  SEXS/1(Efd) -> Efd/1

== system Scenario_1/G1/Speed Governor ==
  note: mechanical power
  RefL : Inport
  dw : Inport  Port=2
  Gain1 : Gain  Gain=Dt
  Gain2 : Gain  Gain=1/R
  Saturation : Saturate  UpperLimit=Vmax  LowerLimit=Vmin
  Saturation1 : Saturate  UpperLimit=1
  Sum : Sum  Inputs=|+-
  Sum1 : Sum  Inputs=|+-
  Transfer Fcn (with initial outputs)1 : simulink_extras/Additional Linear/Transfer Fcn (with initial outputs)  N=[T2 1]  D=[T3 1]  Y0=P0  U0=P0
  Transfer Fcn (with initial outputs)2 : simulink_extras/Additional Linear/Transfer Fcn (with initial outputs)  N=[1]  D=[T1 1]  Y0=P0  U0=P0
  Pm : Outport
  wires:
  Saturation1/1 -> Pm/1
  RefL/1 -> Sum/1
  Sum/1 -> Transfer Fcn (with initial outputs)2/1
  Transfer Fcn (with initial outputs)2/1 -> Saturation/1
  Saturation/1 -> Transfer Fcn (with initial outputs)1/1
  Sum1/1 -> Saturation1/1
  Transfer Fcn (with initial outputs)1/1 -> Sum1/1
  Gain1/1 -> Sum1/2
  dw/1 -> Gain1/1, Gain2/1
  Gain2/1 -> Sum/2

== system Scenario_1/G2/VSC ==
  note: If using different transformer connection,
      | compensate the delay in the modulation
  Block : Step  Time=tonvsc  Before=1  After=0  SampleTime=0
  NOT : Logic  Operator=NOT  IconShape=distinctive  AllPortsSameDT=off  OutDataTypeStr=boolean
  Pset : Step  Time=tonvsc  After=-S2non*G2gen  SampleTime=0
  Qset : Step  Time=tonvsc  After=-30e6  SampleTime=0
  Three-Phase Transformer (Two Windings) : powerlib/Elements/Three-Phase Transformer (Two Windings)  Winding1Connection=Yg  Winding2Connection=Delta (D11)  CoreType=Three single-phase transformers  SetSaturation=off  Hysteresis=off  DataFile='hysteresis'  SetInitialFlux=off  Measurements=None  UNITS=pu  NominalPower=[Pconv , fg ]  Winding1=[Vhv, Rtpu/2, Xtpu/2]  Winding2=[Vmv, Rtpu/2, Xtpu/2]  Rm=5000  Lm=5000  L0=0.5  Saturation=[ 0,0 ; 0.0024,1.2 ; 1.0,1.52 ]  InitialFluxes=[ 0.8 , -0.8 , 0.7 ]  BreakLoop=off  DiscreteSolver=Trapezoidal iterative  DataType=off  TransfoNumber=1
  Three-Phase Breaker : powerlib/Elements/Three-Phase Breaker  InitialState=open  SwitchA=on  SwitchB=on  SwitchC=on  SwitchTimes="[1/60  5/60]"  External=on  BreakerResistance=0.001  SnubberResistance=1e7  SnubberCapacitance=inf  Measurements=None
  VI measurement : Subsystem
      settings: PortSchema="{\"entries\":[{\"content\":{\"sides\":[{\"content\":{\"connectorIds\":[\"LConn1\",\"LConn2\",\"LConn3\"]},\"type\":\"ConnectorPlacement.EquallySpacedRectSide\",\"uuid\":\"d0d5b0b8-afec-4f90-9eba-536a06b10059\"},{\"content\":{\"connectorIds\":[\"RConn1\",\"RConn2\",\"RConn3\"],\"side\":\"RIGHT\"},\"type\":\"ConnectorPlacement.EquallySpacedRectSide\",\"uuid\":\"adc1b68d-6172-4507-b54b-9373921355a1\"},{\"content\":{\"connectorIds\":[\"Out1\",\"Out2\"],\"side\":\"TOP\"},\"type\":\"ConnectorPlacement.EquallySpacedRectSide\",\"uuid\":\"8c5adf07-e95b-4907-94c3-1b2a47d47f40\"}]},\"type\":\"ConnectorPlacement.EquallySpacedConnector\",\"uuid\":\"87d0b20f-8f85-4790-a611-3415e642a83a\"}],\"packageUris\":[\"http://schema.mathworks.com/mf0/Connector/R2020b\"],\"version\":\"1.0\"}"
  VSC Control : Subsystem
      settings: PortSchema="{\"entries\":[{\"content\":{\"sides\":[{\"content\":{\"connectorIds\":[\"In1\",\"In2\",\"In3\",\"In4\",\"In5\"]},\"type\":\"ConnectorPlacement.EquallySpacedRectSide\",\"uuid\":\"cada8d9e-53e0-4197-9386-6c7b6ea13844\"},{\"content\":{\"connectorIds\":[\"Out1\"],\"side\":\"RIGHT\"},\"type\":\"ConnectorPlacement.EquallySpacedRectSide\",\"uuid\":\"f237b52a-0d77-45c0-937d-32cafba1283e\"},{\"content\":{\"connectorIds\":[\"Out2\"],\"side\":\"TOP\"},\"type\":\"ConnectorPlacement.EquallySpacedRectSide\",\"uuid\":\"e6f268b5-5f09-49a6-9529-b1aeebd5f021\"}]},\"type\":\"ConnectorPlacement.EquallySpacedConnector\",\"uuid\":\"4d1d2957-2eb9-4111-8c87-957e800b2b0b\"}],\"packageUris\":[\"http://schema.mathworks.com/mf0/Connector/19700101\"],\"version\":\"1.0\"}"
  VSC Model : Subsystem  Variant=on  VariantControlMode=label  LabelModeActiveChoice=Phasor
      settings: PortSchema="{\"entries\":[{\"content\":{\"sides\":[{\"content\":{\"connectorIds\":[\"LConn1\",\"LConn2\",\"LConn3\"]},\"type\":\"ConnectorPlacement.EquallySpacedRectSide\",\"uuid\":\"96043b84-a665-4cb2-a938-d6633d7ee474\"},{\"content\":{\"connectorIds\":[\"In1\"],\"side\":\"RIGHT\"},\"type\":\"ConnectorPlacement.EquallySpacedRectSide\",\"uuid\":\"064d463f-c23a-42ac-89ce-8dea3d446214\"},{\"content\":{\"connectorIds\":[],\"side\":\"TOP\"},\"type\":\"ConnectorPlacement.EquallySpacedRectSide\",\"uuid\":\"95ef669c-c6ed-44c3-8b69-447906728b6d\"}]},\"type\":\"ConnectorPlacement.EquallySpacedConnector\",\"uuid\":\"ea66db09-64d7-4d7e-ba7b-d769c56e2dbd\"}],\"packageUris\":[\"http://schema.mathworks.com/mf0/Connector/19700101\"],\"version\":\"1.0\"}"
  output signals : Subsystem
  A : PMIOPort  Side=Left
  B : PMIOPort  Port=2  Side=Left
  C : PMIOPort  Port=3  Side=Left
  m : Outport
  wires:
  NOT/1 -> Three-Phase Breaker/1
  VSC Control/1(Ref) -> VSC Model/1(Ref)
  [Is] -> VSC Control/3(Iabc)
  [Vs] -> VSC Control/2(Vabc)
  Block/1 -> VSC Control/1(Block), NOT/1
  [Vs] -> output signals/1(Vs)
  [Is] -> output signals/2(Is)
  VSC Control/2(m) -> output signals/3(control)
  output signals/1(m) -> m/1
  VI measurement/1(Vs) -> [Vs]
  VI measurement/2(Is) -> [Is]
  Pset/1 -> VSC Control/4(Pset)
  Qset/1 -> VSC Control/5(Qset)
  connections:
  Three-Phase Transformer (Two Windings)/LConn3 -- Three-Phase Breaker/LConn3
  Three-Phase Transformer (Two Windings)/LConn2 -- Three-Phase Breaker/LConn2
  Three-Phase Transformer (Two Windings)/LConn1 -- Three-Phase Breaker/LConn1
  Three-Phase Transformer (Two Windings)/RConn3 -- VSC Model/LConn3
  Three-Phase Transformer (Two Windings)/RConn2 -- VSC Model/LConn2
  Three-Phase Transformer (Two Windings)/RConn1 -- VSC Model/LConn1
  Three-Phase Breaker/RConn1 -- VI measurement/RConn1
  Three-Phase Breaker/RConn2 -- VI measurement/RConn2
  Three-Phase Breaker/RConn3 -- VI measurement/RConn3
  VI measurement/LConn3 -- C/RConn1
  A/RConn1 -- VI measurement/LConn1
  B/RConn1 -- VI measurement/LConn2

== system Scenario_1/G3/VSC ==
  note: If using different transformer connection,
      | compensate the delay in the modulation
  Block : Step  Time=tonvsc  Before=1  After=0  SampleTime=0
  NOT : Logic  Operator=NOT  IconShape=distinctive  AllPortsSameDT=off  OutDataTypeStr=boolean
  Pset : Step  Time=tonvsc  After=-S3non*G3gen  SampleTime=0
  Qset : Step  Time=tonvsc  After=-30e6  SampleTime=0
  Three-Phase Transformer (Two Windings) : powerlib/Elements/Three-Phase Transformer (Two Windings)  Winding1Connection=Yg  Winding2Connection=Delta (D11)  CoreType=Three single-phase transformers  SetSaturation=off  Hysteresis=off  DataFile='hysteresis'  SetInitialFlux=off  Measurements=None  UNITS=pu  NominalPower=[Pconv , fg ]  Winding1=[Vhv, Rtpu/2, Xtpu/2]  Winding2=[Vmv, Rtpu/2, Xtpu/2]  Rm=5000  Lm=5000  L0=0.5  Saturation=[ 0,0 ; 0.0024,1.2 ; 1.0,1.52 ]  InitialFluxes=[ 0.8 , -0.8 , 0.7 ]  BreakLoop=off  DiscreteSolver=Trapezoidal iterative  DataType=off  TransfoNumber=1
  Three-Phase Breaker : powerlib/Elements/Three-Phase Breaker  InitialState=open  SwitchA=on  SwitchB=on  SwitchC=on  SwitchTimes="[1/60  5/60]"  External=on  BreakerResistance=0.001  SnubberResistance=1e7  SnubberCapacitance=inf  Measurements=None
  VI measurement : Subsystem
      settings: PortSchema="{\"entries\":[{\"content\":{\"sides\":[{\"content\":{\"connectorIds\":[\"LConn1\",\"LConn2\",\"LConn3\"]},\"type\":\"ConnectorPlacement.EquallySpacedRectSide\",\"uuid\":\"d0d5b0b8-afec-4f90-9eba-536a06b10059\"},{\"content\":{\"connectorIds\":[\"RConn1\",\"RConn2\",\"RConn3\"],\"side\":\"RIGHT\"},\"type\":\"ConnectorPlacement.EquallySpacedRectSide\",\"uuid\":\"adc1b68d-6172-4507-b54b-9373921355a1\"},{\"content\":{\"connectorIds\":[\"Out1\",\"Out2\"],\"side\":\"TOP\"},\"type\":\"ConnectorPlacement.EquallySpacedRectSide\",\"uuid\":\"8c5adf07-e95b-4907-94c3-1b2a47d47f40\"}]},\"type\":\"ConnectorPlacement.EquallySpacedConnector\",\"uuid\":\"87d0b20f-8f85-4790-a611-3415e642a83a\"}],\"packageUris\":[\"http://schema.mathworks.com/mf0/Connector/R2020b\"],\"version\":\"1.0\"}"
  VSC Control : Subsystem
      settings: PortSchema="{\"entries\":[{\"content\":{\"sides\":[{\"content\":{\"connectorIds\":[\"In1\",\"In2\",\"In3\",\"In4\",\"In5\"]},\"type\":\"ConnectorPlacement.EquallySpacedRectSide\",\"uuid\":\"cada8d9e-53e0-4197-9386-6c7b6ea13844\"},{\"content\":{\"connectorIds\":[\"Out1\"],\"side\":\"RIGHT\"},\"type\":\"ConnectorPlacement.EquallySpacedRectSide\",\"uuid\":\"f237b52a-0d77-45c0-937d-32cafba1283e\"},{\"content\":{\"connectorIds\":[\"Out2\"],\"side\":\"TOP\"},\"type\":\"ConnectorPlacement.EquallySpacedRectSide\",\"uuid\":\"e6f268b5-5f09-49a6-9529-b1aeebd5f021\"}]},\"type\":\"ConnectorPlacement.EquallySpacedConnector\",\"uuid\":\"4d1d2957-2eb9-4111-8c87-957e800b2b0b\"}],\"packageUris\":[\"http://schema.mathworks.com/mf0/Connector/19700101\"],\"version\":\"1.0\"}"
  VSC Model : Subsystem  Variant=on  VariantControlMode=label  LabelModeActiveChoice=Phasor
      settings: PortSchema="{\"entries\":[{\"content\":{\"sides\":[{\"content\":{\"connectorIds\":[\"LConn1\",\"LConn2\",\"LConn3\"]},\"type\":\"ConnectorPlacement.EquallySpacedRectSide\",\"uuid\":\"96043b84-a665-4cb2-a938-d6633d7ee474\"},{\"content\":{\"connectorIds\":[\"In1\"],\"side\":\"RIGHT\"},\"type\":\"ConnectorPlacement.EquallySpacedRectSide\",\"uuid\":\"064d463f-c23a-42ac-89ce-8dea3d446214\"},{\"content\":{\"connectorIds\":[],\"side\":\"TOP\"},\"type\":\"ConnectorPlacement.EquallySpacedRectSide\",\"uuid\":\"95ef669c-c6ed-44c3-8b69-447906728b6d\"}]},\"type\":\"ConnectorPlacement.EquallySpacedConnector\",\"uuid\":\"ea66db09-64d7-4d7e-ba7b-d769c56e2dbd\"}],\"packageUris\":[\"http://schema.mathworks.com/mf0/Connector/19700101\"],\"version\":\"1.0\"}"
  output signals : Subsystem
  A : PMIOPort  Side=Left
  B : PMIOPort  Port=2  Side=Left
  C : PMIOPort  Port=3  Side=Left
  m : Outport
  wires:
  NOT/1 -> Three-Phase Breaker/1
  VSC Control/1(Ref) -> VSC Model/1(Ref)
  [Is] -> VSC Control/3(Iabc)
  [Vs] -> VSC Control/2(Vabc)
  Block/1 -> VSC Control/1(Block), NOT/1
  [Vs] -> output signals/1(Vs)
  [Is] -> output signals/2(Is)
  VSC Control/2(m) -> output signals/3(control)
  output signals/1(m) -> m/1
  VI measurement/1(Vs) -> [Vs]
  VI measurement/2(Is) -> [Is]
  Pset/1 -> VSC Control/4(Pset)
  Qset/1 -> VSC Control/5(Qset)
  connections:
  Three-Phase Transformer (Two Windings)/LConn3 -- Three-Phase Breaker/LConn3
  Three-Phase Transformer (Two Windings)/LConn2 -- Three-Phase Breaker/LConn2
  Three-Phase Transformer (Two Windings)/LConn1 -- Three-Phase Breaker/LConn1
  Three-Phase Transformer (Two Windings)/RConn3 -- VSC Model/LConn3
  Three-Phase Transformer (Two Windings)/RConn2 -- VSC Model/LConn2
  Three-Phase Transformer (Two Windings)/RConn1 -- VSC Model/LConn1
  Three-Phase Breaker/RConn1 -- VI measurement/RConn1
  Three-Phase Breaker/RConn2 -- VI measurement/RConn2
  Three-Phase Breaker/RConn3 -- VI measurement/RConn3
  VI measurement/LConn3 -- C/RConn1
  A/RConn1 -- VI measurement/LConn1
  B/RConn1 -- VI measurement/LConn2

== system Scenario_1/G5/VSC ==
  note: If using different transformer connection,
      | compensate the delay in the modulation
  Block : Step  Time=tonvsc  Before=1  After=0  SampleTime=0
  NOT : Logic  Operator=NOT  IconShape=distinctive  AllPortsSameDT=off  OutDataTypeStr=boolean
  Pset : Step  Time=tonvsc  After=-S5non*G5gen  SampleTime=0
  Qset : Step  Time=tonvsc  After=-30e6  SampleTime=0
  Three-Phase Transformer (Two Windings) : powerlib/Elements/Three-Phase Transformer (Two Windings)  Winding1Connection=Yg  Winding2Connection=Delta (D11)  CoreType=Three single-phase transformers  SetSaturation=off  Hysteresis=off  DataFile='hysteresis'  SetInitialFlux=off  Measurements=None  UNITS=pu  NominalPower=[Pconv , fg ]  Winding1=[Vhv, Rtpu/2, Xtpu/2]  Winding2=[Vmv, Rtpu/2, Xtpu/2]  Rm=5000  Lm=5000  L0=0.5  Saturation=[ 0,0 ; 0.0024,1.2 ; 1.0,1.52 ]  InitialFluxes=[ 0.8 , -0.8 , 0.7 ]  BreakLoop=off  DiscreteSolver=Trapezoidal iterative  DataType=off  TransfoNumber=1
  Three-Phase Breaker : powerlib/Elements/Three-Phase Breaker  InitialState=open  SwitchA=on  SwitchB=on  SwitchC=on  SwitchTimes="[1/60  5/60]"  External=on  BreakerResistance=0.001  SnubberResistance=1e7  SnubberCapacitance=inf  Measurements=None
  VI measurement : Subsystem
      settings: PortSchema="{\"entries\":[{\"content\":{\"sides\":[{\"content\":{\"connectorIds\":[\"LConn1\",\"LConn2\",\"LConn3\"]},\"type\":\"ConnectorPlacement.EquallySpacedRectSide\",\"uuid\":\"d0d5b0b8-afec-4f90-9eba-536a06b10059\"},{\"content\":{\"connectorIds\":[\"RConn1\",\"RConn2\",\"RConn3\"],\"side\":\"RIGHT\"},\"type\":\"ConnectorPlacement.EquallySpacedRectSide\",\"uuid\":\"adc1b68d-6172-4507-b54b-9373921355a1\"},{\"content\":{\"connectorIds\":[\"Out1\",\"Out2\"],\"side\":\"TOP\"},\"type\":\"ConnectorPlacement.EquallySpacedRectSide\",\"uuid\":\"8c5adf07-e95b-4907-94c3-1b2a47d47f40\"}]},\"type\":\"ConnectorPlacement.EquallySpacedConnector\",\"uuid\":\"87d0b20f-8f85-4790-a611-3415e642a83a\"}],\"packageUris\":[\"http://schema.mathworks.com/mf0/Connector/R2020b\"],\"version\":\"1.0\"}"
  VSC Control : Subsystem
      settings: PortSchema="{\"entries\":[{\"content\":{\"sides\":[{\"content\":{\"connectorIds\":[\"In1\",\"In2\",\"In3\",\"In4\",\"In5\"]},\"type\":\"ConnectorPlacement.EquallySpacedRectSide\",\"uuid\":\"cada8d9e-53e0-4197-9386-6c7b6ea13844\"},{\"content\":{\"connectorIds\":[\"Out1\"],\"side\":\"RIGHT\"},\"type\":\"ConnectorPlacement.EquallySpacedRectSide\",\"uuid\":\"f237b52a-0d77-45c0-937d-32cafba1283e\"},{\"content\":{\"connectorIds\":[\"Out2\"],\"side\":\"TOP\"},\"type\":\"ConnectorPlacement.EquallySpacedRectSide\",\"uuid\":\"e6f268b5-5f09-49a6-9529-b1aeebd5f021\"}]},\"type\":\"ConnectorPlacement.EquallySpacedConnector\",\"uuid\":\"4d1d2957-2eb9-4111-8c87-957e800b2b0b\"}],\"packageUris\":[\"http://schema.mathworks.com/mf0/Connector/19700101\"],\"version\":\"1.0\"}"
  VSC Model : Subsystem  Variant=on  VariantControlMode=label  LabelModeActiveChoice=Phasor
      settings: PortSchema="{\"entries\":[{\"content\":{\"sides\":[{\"content\":{\"connectorIds\":[\"LConn1\",\"LConn2\",\"LConn3\"]},\"type\":\"ConnectorPlacement.EquallySpacedRectSide\",\"uuid\":\"96043b84-a665-4cb2-a938-d6633d7ee474\"},{\"content\":{\"connectorIds\":[\"In1\"],\"side\":\"RIGHT\"},\"type\":\"ConnectorPlacement.EquallySpacedRectSide\",\"uuid\":\"064d463f-c23a-42ac-89ce-8dea3d446214\"},{\"content\":{\"connectorIds\":[],\"side\":\"TOP\"},\"type\":\"ConnectorPlacement.EquallySpacedRectSide\",\"uuid\":\"95ef669c-c6ed-44c3-8b69-447906728b6d\"}]},\"type\":\"ConnectorPlacement.EquallySpacedConnector\",\"uuid\":\"ea66db09-64d7-4d7e-ba7b-d769c56e2dbd\"}],\"packageUris\":[\"http://schema.mathworks.com/mf0/Connector/19700101\"],\"version\":\"1.0\"}"
  output signals : Subsystem
  A : PMIOPort  Side=Left
  B : PMIOPort  Port=2  Side=Left
  C : PMIOPort  Port=3  Side=Left
  m : Outport
  wires:
  NOT/1 -> Three-Phase Breaker/1
  VSC Control/1(Ref) -> VSC Model/1(Ref)
  [Is] -> VSC Control/3(Iabc)
  [Vs] -> VSC Control/2(Vabc)
  Block/1 -> VSC Control/1(Block), NOT/1
  [Vs] -> output signals/1(Vs)
  [Is] -> output signals/2(Is)
  VSC Control/2(m) -> output signals/3(control)
  output signals/1(m) -> m/1
  VI measurement/1(Vs) -> [Vs]
  VI measurement/2(Is) -> [Is]
  Pset/1 -> VSC Control/4(Pset)
  Qset/1 -> VSC Control/5(Qset)
  connections:
  Three-Phase Transformer (Two Windings)/LConn3 -- Three-Phase Breaker/LConn3
  Three-Phase Transformer (Two Windings)/LConn2 -- Three-Phase Breaker/LConn2
  Three-Phase Transformer (Two Windings)/LConn1 -- Three-Phase Breaker/LConn1
  Three-Phase Transformer (Two Windings)/RConn3 -- VSC Model/LConn3
  Three-Phase Transformer (Two Windings)/RConn2 -- VSC Model/LConn2
  Three-Phase Transformer (Two Windings)/RConn1 -- VSC Model/LConn1
  Three-Phase Breaker/RConn1 -- VI measurement/RConn1
  Three-Phase Breaker/RConn2 -- VI measurement/RConn2
  Three-Phase Breaker/RConn3 -- VI measurement/RConn3
  VI measurement/LConn3 -- C/RConn1
  A/RConn1 -- VI measurement/LConn1
  B/RConn1 -- VI measurement/LConn2
